simulink model "rover_2d_sysid"  (R2021a)
settings: Solver=ode23t  StartTime=0.0  StopTime=30  RelTol=1e-3
values from neighbouring files (symbols this model uses):
  h = 0.2    [Apollo_LM_design_discrete_observer.m]    (also in Apollo_LM_design_observer.m = 0.25; Apollo_LM_state_feedback.m = 0.5)
  s = tf('s')    [Apollo_LM_design_discrete_observer.m]    (also in elastic_shaft_rlocus.m; harmonic_osc_rlocus.m)
undefined symbols (not defined in the file or in its folder): X, Y, Z
libraries: sm_lib x73, nesl_utility x18
(part 1 of 2)
settings Model: Creator=kjartan  LastModifiedBy=kjartan

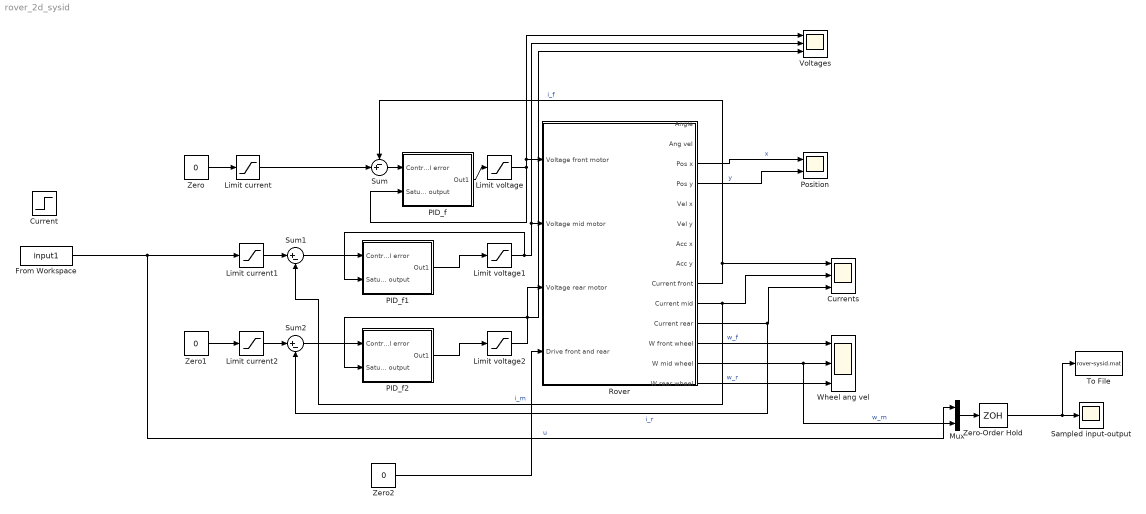
== system rover_2d_sysid ==
  Current : Step  Time=5  After=2e-2  SampleTime=0
  Currents : Scope  NumInputPorts=3
  From Workspace : FromWorkspace  VariableName=input1
  Limit current : Saturate  UpperLimit=10  LowerLimit=-10
  Limit current1 : Saturate  UpperLimit=10  LowerLimit=-10
  Limit current2 : Saturate  UpperLimit=10  LowerLimit=-10
  Limit voltage : Saturate  UpperLimit=48  LowerLimit=-48
  Limit voltage1 : Saturate  UpperLimit=48  LowerLimit=-48
  Limit voltage2 : Saturate  UpperLimit=48  LowerLimit=-48
  Mux : Mux  Inputs=2
  PID_f : Subsystem
  PID_f1 : Subsystem
  PID_f2 : Subsystem
  Position : Scope  NumInputPorts=2
  Rover : Subsystem
  Sampled input-output : Scope
  Sum : Sum  Inputs=-+|
  Sum1 : Sum  Inputs=|+-
  Sum2 : Sum  Inputs=|+-
  To File : ToFile  Filename=rover-sysid.mat  MatrixName=out  SaveFormat=Timeseries
  Voltages : Scope  NumInputPorts=3
  Wheel ang vel : Scope  NumInputPorts=3
  Zero : Constant  Value=0  OutDataTypeStr=Inherit: Inherit via back propagation
  Zero-Order Hold : ZeroOrderHold  SampleTime=h
  Zero1 : Constant  Value=0  OutDataTypeStr=Inherit: Inherit via back propagation
  Zero2 : Constant  Value=0  OutDataTypeStr=Inherit: Inherit via back propagation
  wires:
  Rover/3(Pos x) -> Position/1  "x"
  Rover/9(Current front) -> Sum/1, Currents/1  "i_f"
  Rover/4(Pos y) -> Position/2  "y"
  Rover/12(W front wheel) -> Wheel ang vel/1  "w_f"
  Rover/13(W mid wheel) -> Mux/2, Wheel ang vel/2  "w_m"
  Rover/14(W rear wheel) -> Wheel ang vel/3  "w_r"
  Limit current/1 -> Sum/2
  Limit voltage/1 -> Voltages/1, Rover/1(Voltage front motor), PID_f/2(Saturated output)
  Limit voltage1/1 -> Voltages/2, Rover/2(Voltage mid motor), PID_f1/2(Saturated output)
  Sum1/1 -> PID_f1/1(Control error)
  PID_f1/1(Out1) -> Limit voltage1/1
  Rover/10(Current mid) -> Sum1/2, Currents/2  "i_m"
  Limit current1/1 -> Sum1/1
  Limit voltage2/1 -> Rover/3(Voltage rear motor), Voltages/3, PID_f2/2(Saturated output)
  Sum2/1 -> PID_f2/1(Control error)
  PID_f2/1(Out1) -> Limit voltage2/1
  Rover/11(Current rear) -> Sum2/2, Currents/3  "i_r"
  Limit current2/1 -> Sum2/1
  From Workspace/1 -> Mux/1, Limit current1/1  "u"
  Sum/1 -> PID_f/1(Control error)
  PID_f/1(Out1) -> Limit voltage/1
  Zero/1 -> Limit current/1
  Zero1/1 -> Limit current2/1
  Zero-Order Hold/1 -> To File/1, Sampled input-output/1
  Mux/1 -> Zero-Order Hold/1
  Zero2/1 -> Rover/4(Drive front and rear)

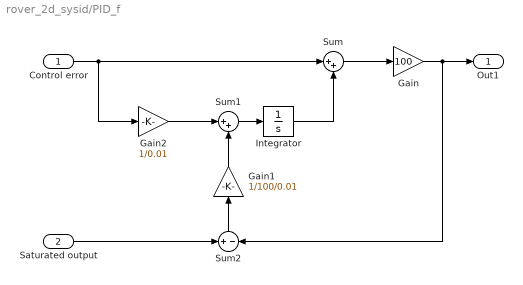
== system rover_2d_sysid/PID_f ==
  Control error : Inport
  Saturated output : Inport  Port=2
  Gain : Gain  Gain=100
  Gain1 : Gain  Gain=1/100/0.01
  Gain2 : Gain  Gain=1/0.01
  Integrator : Integrator
  Sum : Sum  Inputs=|++
  Sum1 : Sum  Inputs=|++
  Sum2 : Sum  Inputs=+|-
  Out1 : Outport
  wires:
  Control error/1 -> Gain2/1, Sum/1
  Gain/1 -> Sum2/2, Out1/1
  Sum/1 -> Gain/1
  Saturated output/1 -> Sum2/1
  Sum2/1 -> Gain1/1
  Gain1/1 -> Sum1/2
  Sum1/1 -> Integrator/1
  Integrator/1 -> Sum/2
  Gain2/1 -> Sum1/1

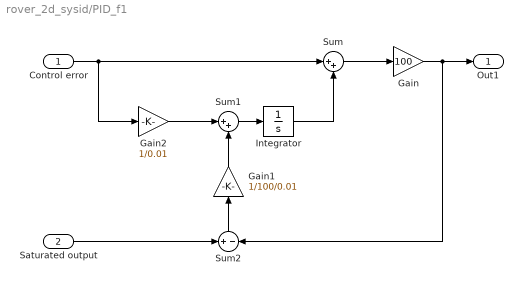
== system rover_2d_sysid/PID_f1 ==
  Control error : Inport
  Saturated output : Inport  Port=2
  Gain : Gain  Gain=100
  Gain1 : Gain  Gain=1/100/0.01
  Gain2 : Gain  Gain=1/0.01
  Integrator : Integrator
  Sum : Sum  Inputs=|++
  Sum1 : Sum  Inputs=|++
  Sum2 : Sum  Inputs=+|-
  Out1 : Outport
  wires:
  Control error/1 -> Gain2/1, Sum/1
  Gain/1 -> Sum2/2, Out1/1
  Sum/1 -> Gain/1
  Saturated output/1 -> Sum2/1
  Sum2/1 -> Gain1/1
  Gain1/1 -> Sum1/2
  Sum1/1 -> Integrator/1
  Integrator/1 -> Sum/2
  Gain2/1 -> Sum1/1

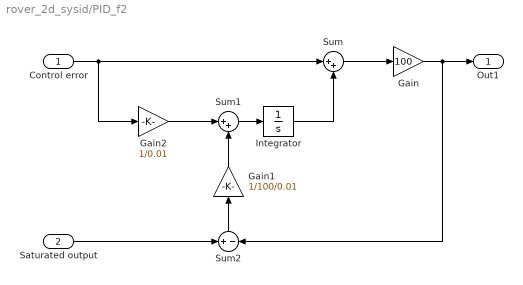
== system rover_2d_sysid/PID_f2 ==
  Control error : Inport
  Saturated output : Inport  Port=2
  Gain : Gain  Gain=100
  Gain1 : Gain  Gain=1/100/0.01
  Gain2 : Gain  Gain=1/0.01
  Integrator : Integrator
  Sum : Sum  Inputs=|++
  Sum1 : Sum  Inputs=|++
  Sum2 : Sum  Inputs=+|-
  Out1 : Outport
  wires:
  Control error/1 -> Gain2/1, Sum/1
  Gain/1 -> Sum2/2, Out1/1
  Sum/1 -> Gain/1
  Saturated output/1 -> Sum2/1
  Sum2/1 -> Gain1/1
  Gain1/1 -> Sum1/2
  Sum1/1 -> Integrator/1
  Integrator/1 -> Sum/2
  Gain2/1 -> Sum1/1
